simulink model "jietu"  (Simulink 8.3)
settings: Solver=ode45  StartTime=0.0  StopTime=15  RelTol=1e-3
undefined symbols (not defined in the file or in its folder): gay, sigbuilder_block
libraries: Solver_SF x1
settings Model: Creator=win8  LastModifiedBy=yzhnu
settings OptimizationCC: ExpressionDepthLimit=2147483647
settings DebuggingCC: FcnCallInpInsideContextMsg=UseLocalSettings

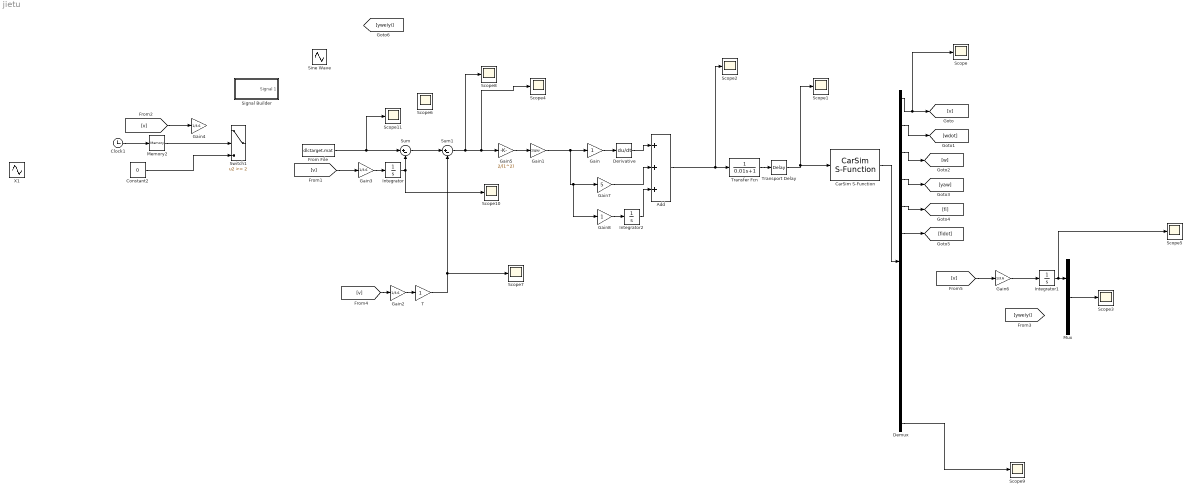
== system jietu ==
  Add : Sum  Inputs=+++
  CarSim S-Function : Solver_SF/CarSim S-Function  Priority=1  VehicleCode=i_s  SIMFILE=simfile
  Clock1 : Clock
  Constant2 : Constant  Value=0
  Demux : Demux  Outputs=13
  Derivative : Derivative
  From File : FromFile  FileName=dlctarget.mat  SampleTime=0
  Gain : Gain
  Gain1 : Gain  Gain=1/gay
  Gain{2..4,6} (4 alike) : Gain  Gain=1/3.6
  Gain5 : Gain  Gain=2/(1^2)
  Gain7 : Gain  Gain=5
  Gain8 : Gain
  Integrator : Integrator
  Integrator1 : Integrator
  Integrator2 : Integrator
  Memory2 : Memory
  Mux : Mux  Inputs=2
  Scope{,1..11} (12 alike) : Scope
      Scope settings: YMin=-0.5
      Scope1 settings: YMin=-350  YMax=350
      Scope10 settings: YMin=-32.5  YMax=2.5  SaveName=ScopeData10
      Scope11 settings: YMin=0  YMax=3.5  SaveName=ScopeData11
      Scope2 settings: YMin=-900  YMax=400  SaveName=ScopeData2
      Scope3 settings: YMin=-0.5  SaveName=ScopeData3
      Scope4 settings: YMin=0  YMax=3.25  SaveName=ScopeData4
      Scope5 settings: YMin=-0.235  YMax=-0.1975  SaveName=ScopeData5
      Scope6 settings: YMin=0.25  YMax=3.5  SaveName=ScopeData6
      Scope7 settings: YMin=-0.0325  YMax=0  SaveName=ScopeData7
      Scope8 settings: YMin=-200  YMax=25  SaveName=ScopeData8
      Scope9 settings: YMin=0  YMax=3.5  SaveName=ScopeData9
  Signal Builder : Subsystem  Tag=STV Subsys  LoadFcn=sigbuilder_block('load');  StartFcn=sigbuilder_block('start');  StopFcn=sigbuilder_block('stop');  ClipboardFcn=sigbuilder_block('clipboard');  mask(Sigbuilder block){}
      mask help: Simulink:masks:SigbuilderBlock_MD
      mask init:
      | if ~strcmp(get_param(bdroot(gcbh),'SimulationStatus'),'stopped') tuvar = sigbuilder_block('maskInit'); end
      settings: CopyFcn=sigbuilder_block('copy');  DeleteFcn=sigbuilder_block('delete');  ModelCloseFcn=sigbuilder_block('modelClose');  PreSaveFcn=sigbuilder_block('preSave');  PauseFcn=sigbuilder_block('pause');  ContinueFcn=sigbuilder_block('continue');  NameChangeFcn=sigbuilder_block('namechange');  OpenFcn=sigbuilder_block('open',[259.5 113.25 550.5 393.75 ]);  CloseFcn=sigbuilder_block('close');
      mask Display: plot(0, 0, 100, 100,[2, 2, 32, 32, 2], [68, 8, 8, 68, 68],[32, 2], [38, 38], [32, 19, 2],[53, 60, 44], [32, 17, 17, 2],[16, 16, 31, 31]);txt = getActiveGroup(gcbh);text(2, 100, txt,'verticalAlignment', 'top');
  Sine Wave : Sin  Amplitude=3.5  Frequency=0.5  SampleTime=0
  Sum : Sum  Inputs=|+-
  Sum1 : Sum  Inputs=|+-
  Switch1 : Switch  Threshold=2
  T : Gain
  Transfer Fcn : TransferFcn  Denominator=[0.01 1]
  Transport Delay : TransportDelay  DelayTime=0.001
  X1 : Sin  Amplitude=100  SampleTime=0
  wires:
  Sum/1 -> Sum1/1
  Sum1/1 -> Gain5/1, Scope4/1, Scope8/1
  CarSim S-Function/1 -> Demux/1
  Demux/1 -> Scope/1, [v]
  Demux/2 -> [wdot]
  Demux/3 -> [w]
  Demux/4 -> [yaw]
  Demux/5 -> [fi]
  Demux/6 -> [fidot]
  [v] -> Gain3/1
  [v] -> Gain2/1
  Gain2/1 -> T/1
  [v] -> Gain4/1
  Clock1/1 -> Memory2/1
  Memory2/1 -> Switch1/2
  Constant2/1 -> Switch1/3
  Gain3/1 -> Integrator/1
  Integrator/1 -> Scope10/1, Sum/2
  T/1 -> Scope7/1, Sum1/2
  Gain/1 -> Derivative/1
  Derivative/1 -> Add/1
  Gain1/1 -> Gain8/1, Gain7/1, Gain/1
  Add/1 -> Scope2/1, Transfer Fcn/1
  Gain5/1 -> Gain1/1
  Transfer Fcn/1 -> Transport Delay/1
  Transport Delay/1 -> CarSim S-Function/1, Scope1/1
  Mux/1 -> Scope3/1
  [v] -> Gain6/1
  Integrator1/1 -> Scope5/1, Mux/1
  Gain6/1 -> Integrator1/1
  Demux/13 -> Scope9/1
  From File/1 -> Scope11/1, Sum/1
  Gain7/1 -> Add/2
  Gain8/1 -> Integrator2/1
  Integrator2/1 -> Add/3

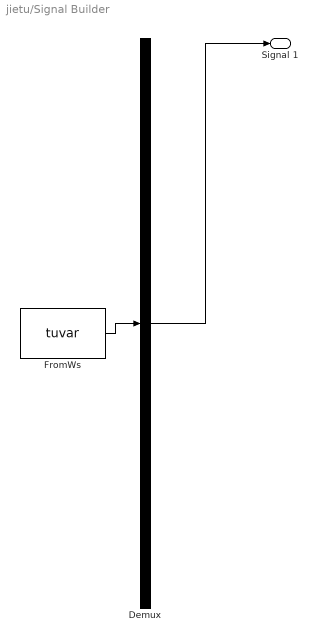
== system jietu/Signal Builder ==
  Demux : Demux  Tag=STV Demux  Outputs=1
  FromWs : FromWorkspace  Tag=STV FromWs  VariableName=tuvar  SampleTime=0  SigBuilderData=DataTag0  VnvData=DataTag1
      SigBuilderData=|
      | common.afterFinalStr = 'Extrapolate'
      | common.sampleTime = 0
      | dataSet.timeRange = [0 10]
      | dataSet.name = 'Group 1'
      | sbobj.Groups.Name = 'Group 1'
      | sbobj.Groups.Signals.Name = 'Signal 1'
      | sbobj.Groups.Signals.XData = [0 3.5 4 6 6.5 10]
      | sbobj.Groups.Signals.YData = [0 0 3.5 3.5 0 0]
  Signal 1 : Outport  Tag=STV Outport
  wires:
  Demux/1 -> Signal 1/1
  FromWs/1 -> Demux/1
